simulink model "aa1"  (R2012b)
settings: Solver=ode45  StartTime=0.0  StopTime=10.0  RelTol=1e-3
settings Model: Creator=Administrator  LastModifiedBy=Administrator

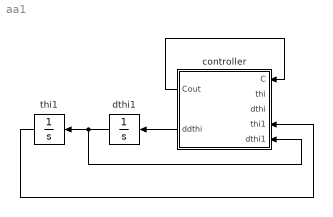
== system aa1 ==
  controller : MATLAB Function  TreatAsAtomicUnit=on
  dthi1 : Integrator
  thi1 : Integrator
  wires:
  controller/2(ddthi) -> dthi1/1
  dthi1/1 -> controller/5(dthi1), thi1/1
  thi1/1 -> controller/4(thi1)
  controller/1(Cout) -> controller/1(C)

== matlab function aa1/controller ==
  data: C input; thi input; dthi input; thi1 input; dthi1 input; Cout output; ddthi output
function [Cout, ddthi] = fcn(C, thi, dthi, thi1, dthi1)
Mp = 135;
Mr = 5.5;
D = 0.6;
L = 1;
b = 0.03;
R = 0.2;
Jp = 27.6;
Jr = 0.11;
g = 9.8;

%**************************************************************************
%线性模型
%**************************************************************************
alpha = Mr * R ^ 2 / Jr + 1;
beta = Jp / (Mp * L) + L;
gama = L * Mp * g;
A22 = -R ^ 2 * b / (alpha * Jr);
A23 = -R ^ 2 * gama / (2 * Jr * alpha * beta);
B2 = R / (2 * Jr) * (1 / alpha + R / (alpha * beta));
A43 = gama / Jp - (L * gama) / (Jp * beta);
B4 = (L / beta - 1) / Jp;
%**************************************************************************
%dthi = dthi + 1227400 * (thi - thi1) + 430300 * (dthi - dthi1);
ddthi = A43 * thi + B4 * C + 430300 * (thi - thi1) + 150800 * (dthi - dthi1);
Cout = 2646 * thi1 + 927 * dthi1;
